simulink model "arinc"  (R2018b)
settings: Solver=FixedStepAuto  StartTime=0.0  StopTime=30  RelTol=1e-3
libraries: sldvlib x10, simulink x2
settings Model: Creator=natppu  LastModifiedBy=natppu
settings ConfigComp: DVTestSuiteOptimization=CombinedObjectives (Nonlinear Extended)  DVDetectOutOfBounds=on  DVProvingStrategy=ProveWithViolationDetection  DVMaxViolationSteps=30

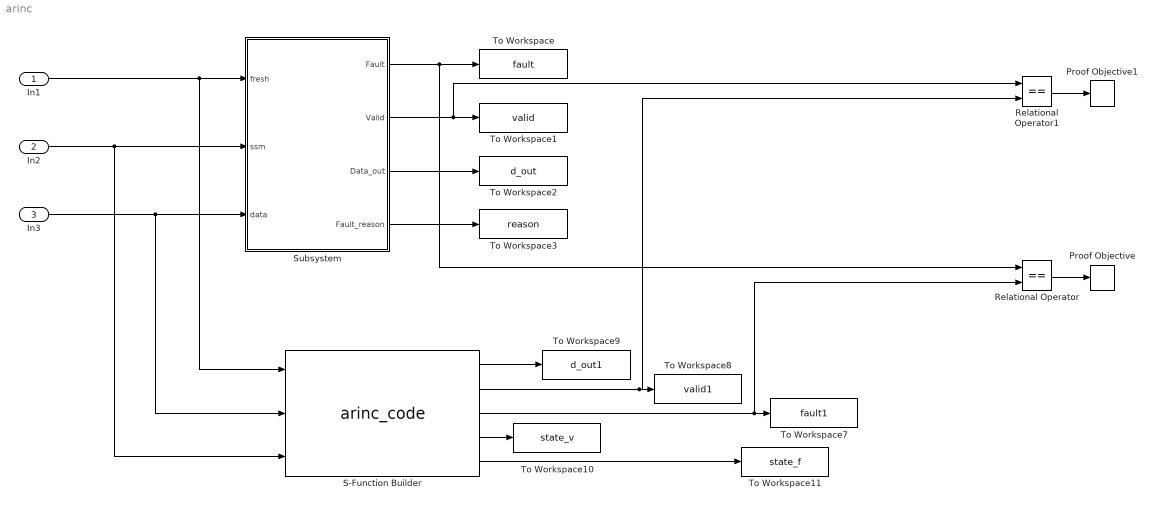
== system arinc ==
  In1 : Inport  OutDataTypeStr=boolean
  In2 : Inport  Port=2  OutMin=1  OutMax=4  OutDataTypeStr=int32
  In3 : Inport  Port=3  OutDataTypeStr=int32
  Proof Objective : sldvlib/Objectives and Constraints/Proof Objective  enabled=on  customAVTBlockType=Proof Objective  intervals=true  dispValues=on  outEnabled=off  enableStopSim=off
      settings: AttributesFormatString=%<intervals>  SourceProductName=Simulink Design Verifier  SourceProductBaseCode=DV
  Proof Objective1 : sldvlib/Objectives and Constraints/Proof Objective  enabled=on  customAVTBlockType=Proof Objective  intervals=true  dispValues=on  outEnabled=off  enableStopSim=off
      settings: AttributesFormatString=%<intervals>  SourceProductName=Simulink Design Verifier  SourceProductBaseCode=DV
  Relational Operator : RelationalOperator  Operator===  OutDataTypeStr=boolean  RndMeth=Simplest
  Relational Operator1 : RelationalOperator  Operator===  OutDataTypeStr=boolean  RndMeth=Simplest
  S-Function Builder : S-Function  InitFcn=try, set_param(gcb,'FunctionName','arinc_code'), end  FunctionName=arinc_code  SFunctionModules=arinc_code_wrapper  SFunctionDeploymentMode=off  EnableBusSupport=off  mask(S-Function Builder){}
      mask help: Simulink:masks:SFunctionBuilder_MD
      mask init:
      | val = [[.9  0.75 0.75 1 1 .9 .9 1]',[1 1 0.75 0.75 .9 .9 1 .9]'];try , sys = get_param(gcb,'SfunBuilderFcnName');if isempty(sys), sys = get_param(gcb,'FunctionName'); end,catch, sys = get_param(gcb,'FunctionName'); end
      settings: CopyFcn=set_param(gcbh,'LinkStatus','none')  PreSaveFcn=try, set_param(gcb,'FunctionName','arinc_code'), end  OpenFcn=sfunctionwizard(gcbh)
      mask Display: plot(val(:,1),val(:,2)),disp(sys), port_label('input',1,'i_fresh'), port_label('input',2,'i_data'), port_label('input',3,'i_ssm'), port_label('output',1,'o_data'), port_label('output',2,'o_valid'), port_label('output',3,'o_fault'), port_label('output',4,'o_state_v'), port_label('output',5,'o_state_f')
  Subsystem : Subsystem  TreatAsAtomicUnit=on
  To Workspace : ToWorkspace  VariableName=fault  SampleTime=-1
      settings: Save2DSignal=2-D array (concatenate along first dimension)
  To Workspace1 : ToWorkspace  VariableName=valid  SampleTime=-1
      settings: Save2DSignal=2-D array (concatenate along first dimension)
  To Workspace10 : ToWorkspace  VariableName=state_v  SampleTime=-1
      settings: Save2DSignal=2-D array (concatenate along first dimension)
  To Workspace11 : ToWorkspace  VariableName=state_f  SampleTime=-1
      settings: Save2DSignal=2-D array (concatenate along first dimension)
  To Workspace2 : ToWorkspace  VariableName=d_out  SampleTime=-1
      settings: Save2DSignal=2-D array (concatenate along first dimension)
  To Workspace3 : ToWorkspace  VariableName=reason  SampleTime=-1
      settings: Save2DSignal=2-D array (concatenate along first dimension)
  To Workspace7 : ToWorkspace  VariableName=fault1  SampleTime=-1
      settings: Save2DSignal=2-D array (concatenate along first dimension)
  To Workspace8 : ToWorkspace  VariableName=valid1  SampleTime=-1
      settings: Save2DSignal=2-D array (concatenate along first dimension)
  To Workspace9 : ToWorkspace  VariableName=d_out1  SampleTime=-1
      settings: Save2DSignal=2-D array (concatenate along first dimension)
  wires:
  Subsystem/1(Fault) -> Relational Operator/1, To Workspace/1
  S-Function Builder/4 -> To Workspace10/1
  Subsystem/4(Fault_reason) -> To Workspace3/1
  S-Function Builder/5 -> To Workspace11/1
  In1/1 -> S-Function Builder/1, Subsystem/1(fresh)
  In2/1 -> S-Function Builder/3, Subsystem/2(ssm)
  In3/1 -> S-Function Builder/2, Subsystem/3(data)
  S-Function Builder/3 -> Relational Operator/2, To Workspace7/1
  Relational Operator/1 -> Proof Objective/1
  Subsystem/2(Valid) -> Relational Operator1/1, To Workspace1/1
  S-Function Builder/2 -> Relational Operator1/2, To Workspace8/1
  Relational Operator1/1 -> Proof Objective1/1
  Subsystem/3("Data_out ") -> To Workspace2/1
  S-Function Builder/1 -> To Workspace9/1

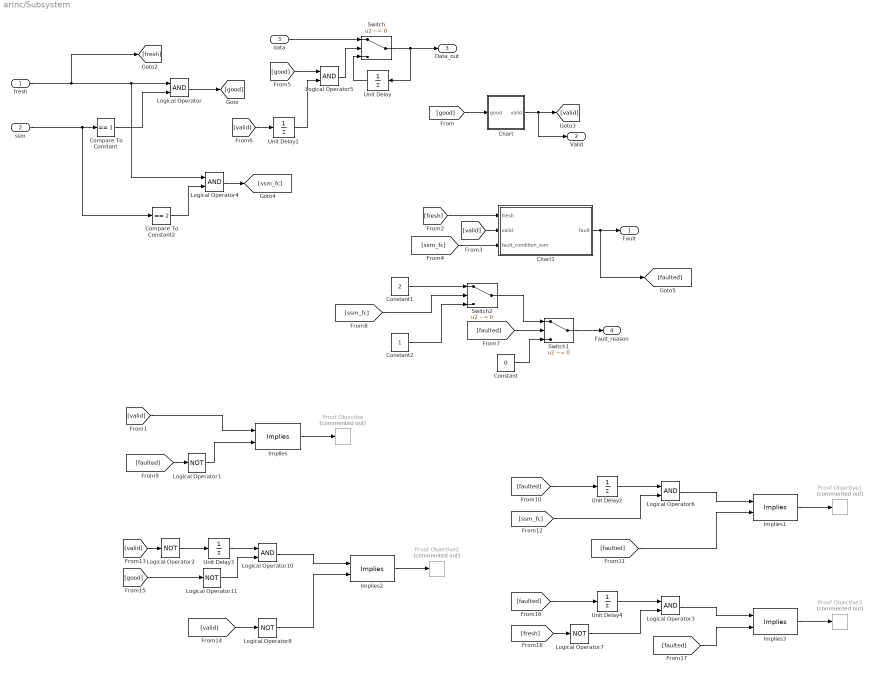
== system arinc/Subsystem ==
  fresh : Inport
  ssm : Inport  Port=2
  data : Inport  Port=3
  Chart : Stateflow chart  TreatAsAtomicUnit=on
  Chart1 : Stateflow chart  TreatAsAtomicUnit=on
  Compare To Constant : simulink/Logic and Bit Operations/Compare To Constant  relop===  const=1  OutDataTypeStr=boolean
  Compare To Constant2 : simulink/Logic and Bit Operations/Compare To Constant  relop===  const=2  OutDataTypeStr=boolean
  Constant : Constant  Value=0  OutDataTypeStr=int32
  Constant1 : Constant  Value=2  OutDataTypeStr=int32
  Constant2 : Constant  OutDataTypeStr=int32
  Implies{,1..3} (4 alike) : sldvlib/Verification Utilities/Implies
      settings: SourceProductName=Simulink  SourceProductBaseCode=SL
  Logical Operator{,3..6,10} (6 alike) : Logic  AllPortsSameDT=off  OutDataTypeStr=boolean
  Logical Operator{1..2,7..8,11} (5 alike) : Logic  Operator=NOT  Inputs=1  AllPortsSameDT=off  OutDataTypeStr=boolean
  Proof Objective{,1..3} (4 alike) : sldvlib/Objectives and Constraints/Proof Objective  Commented=on  enabled=on  customAVTBlockType=Proof Objective  intervals=true  dispValues=on  outEnabled=off  enableStopSim=off
      settings: AttributesFormatString=%<intervals>  SourceProductName=Simulink  SourceProductBaseCode=SL
  Switch : Switch  Criteria=u2 ~= 0
  Switch1 : Switch  Criteria=u2 ~= 0
  Switch2 : Switch  Criteria=u2 ~= 0
  Unit Delay{,1..4} (5 alike) : UnitDelay  SampleTime=-1
  Fault : Outport  VectorParamsAs1DForOutWhenUnconnected=on
  Valid : Outport  Port=2  VectorParamsAs1DForOutWhenUnconnected=on
  "Data_out " : Outport  Port=3  VectorParamsAs1DForOutWhenUnconnected=on
  Fault_reason : Outport  Port=4  VectorParamsAs1DForOutWhenUnconnected=on
  wires:
  Constant/1 -> Switch1/3
  Switch/1 -> "Data_out "/1, Unit Delay/1
  Unit Delay/1 -> Switch/3
  [good] -> Logical Operator5/1
  [faulted] -> Switch1/2
  [ssm_fc] -> Switch2/2
  Chart1/1(fault) -> Fault/1, [faulted]
  Constant2/1 -> Switch2/3
  [valid] -> Chart1/2(valid)
  Switch1/1 -> Fault_reason/1
  fresh/1 -> [fresh], Logical Operator4/1, Logical Operator/1
  Compare To Constant/1 -> Logical Operator/2
  ssm/1 -> Compare To Constant2/1, Compare To Constant/1
  Constant1/1 -> Switch2/1
  Switch2/1 -> Switch1/1
  Chart/1(valid) -> Valid/1, [valid]
  [ssm_fc] -> Chart1/3(fault_condition_ssm)
  [fresh] -> Chart1/1(fresh)
  Logical Operator/1 -> [good]
  Logical Operator4/1 -> [ssm_fc]
  data/1 -> Switch/1
  [good] -> Chart/1(good)
  Compare To Constant2/1 -> Logical Operator4/2
  [valid] -> Unit Delay1/1
  Logical Operator5/1 -> Switch/2
  Unit Delay1/1 -> Logical Operator5/2
  Implies/1 -> Proof Objective/1
  [valid] -> Implies/1
  [faulted] -> Logical Operator1/1
  Logical Operator1/1 -> Implies/2
  [faulted] -> Implies1/2
  Implies1/1 -> Proof Objective1/1
  [faulted] -> Unit Delay2/1
  Unit Delay2/1 -> Logical Operator6/1
  [ssm_fc] -> Logical Operator6/2
  Logical Operator6/1 -> Implies1/1
  Logical Operator10/1 -> Implies2/1
  Logical Operator11/1 -> Logical Operator10/2
  [good] -> Logical Operator11/1
  Unit Delay3/1 -> Logical Operator10/1
  [valid] -> Logical Operator2/1
  Implies2/1 -> Proof Objective2/1
  [valid] -> Logical Operator8/1
  Logical Operator8/1 -> Implies2/2
  Logical Operator2/1 -> Unit Delay3/1
  Logical Operator3/1 -> Implies3/1
  [fresh] -> Logical Operator7/1
  Unit Delay4/1 -> Logical Operator3/1
  [faulted] -> Unit Delay4/1
  Implies3/1 -> Proof Objective3/1
  [faulted] -> Implies3/2
  Logical Operator7/1 -> Logical Operator3/2

== stateflow chart arinc/Subsystem/Chart1 ==
  state count_to_fault
    entry:
    count = 1;
    during:
    count = count+1;
  state Init
    fault = false;
    count = 0;
  state fault_set
    entry:
    fault = true;
    count = 0;
  state count_to_health
    entry:
    count = 1;
    during:
    count = count+1;
  state health_set
    entry:
    fault = false;
    count = 0;
  (default) -> Init
  health_set -> count_to_fault : [~valid && (fault_condition_ssm || ~fresh)]
  count_to_fault -> Init [order 3] : [~fault_condition_ssm]
  Init -> count_to_fault [order 2] : [fault_condition_ssm || ~fresh ]
  Init -> health_set [order 1] : [valid]
  count_to_fault -> health_set [order 1] : [valid]
  count_to_fault -> fault_set [order 2] : [count > 6]
  count_to_health -> fault_set [order 2] : [fault_condition_ssm || ~fresh]
  fault_set -> count_to_health [order 2] : [~fault_condition_ssm]
  fault_set -> health_set [order 1] : [valid]
  count_to_health -> health_set [order 1] : [valid]
  count_to_health -> health_set [order 3] : [[count > 6]]
  data: fault output boolean; fresh input; valid input; fault_condition_ssm input; count local

== stateflow chart arinc/Subsystem/Chart ==
  state bad
    entry:
    count = int32(1);
    during:
    count = count+1;
  state init
    entry:
    valid = false;
    count = int32(0);
  state invalid
    entry:
    valid = false;
    count = int32(0);
  state good
    entry:
    count = int32(1);
    during:
    count = count+1;
  state validity
    entry:
    valid = true;
    count = int32(0);
  (default) -> init
  init -> invalid [order 1] : [~good]
  good -> bad [order 1] : [~good]
  bad -> invalid [order 2] : [count > 2]
  init -> good [order 2]
  bad -> good [order 1] : [good]
  validity -> bad : [~good]
  invalid -> good : [good]
  good -> validity [order 2] : [count > 3]
  data: good input boolean; valid output boolean =true; count local int32 =int32(0)
